simulink model "S2_VCO"  (Simulink 7.9)
settings: Solver=ode3  StartTime=0.0  StopTime=5.999  FixedStep=1/fs  RelTol=1e-3
values from neighbouring files (symbols this model uses):
  fs = fs/10    (= 100000)    [PLL_Parameter.m]
undefined symbols (not defined in the file or in its folder): get
libraries: dspspect3 x1, dspsigops x1, simulink x1, dspsnks4 x1
settings Model: Creator=Administrator  LastModifiedBy=root
settings DebuggingCC: FcnCallInpInsideContextMsg=Use local settings
settings GRTTargetCC: CombineOutputUpdateFcns=off  GRTInterface=on

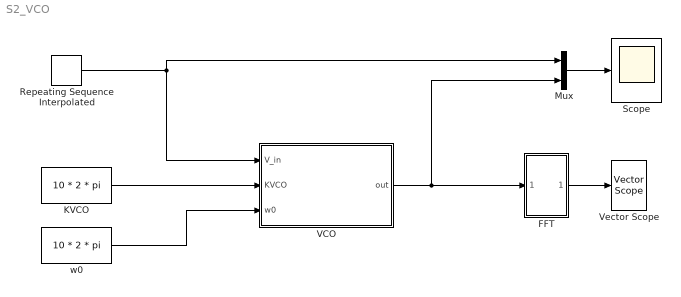
== system S2_VCO ==
  FFT : Subsystem  mask{Buffer_Length=2^14, nfft=2^14}
      mask prompts: Buffer_Length "Buffer length?"; nfft "FFt length?"
  KVCO : Constant  Value=10 * 2 * pi
  Mux : Mux  Inputs=2
  Repeating Sequence Interpolated : simulink/Sources/Repeating Sequence Interpolated  OutValues=[0 0 1 1 -1 -0.9].'  TimeValues=[0 1 3 3.5 5 6].'  LookUpMeth=Interpolation-Use End Values  tsamp=1/fs  OutMin=[]  OutMax=[]  OutDataTypeStr=double  OutputDataTypeScalingMode=double  OutDataType=fixdt(0,8)  OutScaling=2^-10
  Scope : Scope
      settings: TimeRange=1  YMin=-2  YMax=2
  VCO : Subsystem
  Vector Scope : dspsnks4/Vector Scope  ScopeProperties=on  Domain=Frequency  HorizSpan=1  DisplayProperties=off  AxisGrid=on  Memory=off  FrameNumber=on  AxisLegend=off  AxisZoom=off  OpenScopeAtSimStart=on  OpenScopeImmediately=off  FigPos=get(0,'defaultfigureposition')  AxisProperties=off  XUnits=Hertz  XRange=[0...Fs/2]  InheritXIncr=on  XIncr=1  XLabel=Time  XLimit=User-defined  XMin=0  XMax=30  XStart=0  YUnits=dB  YLabel=Amplitude  LineProperties=off  XAxisParamsVer=6.9
      settings: YMin=-100  YMax=100
  w0 : Constant  Value=10 * 2 * pi
  wires:
  VCO/1(out) -> Mux/2, FFT/1(In1)
  w0/1 -> VCO/3(w0)
  KVCO/1 -> VCO/2(KVCO)
  FFT/1(Out1) -> Vector Scope/1
  Repeating Sequence Interpolated/1 -> VCO/1(V_in), Mux/1
  Mux/1 -> Scope/1

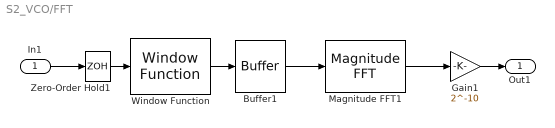
== system S2_VCO/FFT ==
  In1 : Inport
  Buffer1 : Buffer  N=Buffer_Length  TreatMby1Signals=One channel
  Gain1 : Gain  Gain=2^-10
  Magnitude FFT1 : dspspect3/Magnitude FFT  mag_or_magsq=Magnitude squared  FFTImplementation=Auto  fftLenInherit=off  fftsize=nfft
  Window Function : dspsigops/Window Function  winmode=Apply window to input  wintype=Blackman  sampmode=Continuous  samptime=1  N=64  Rs=50  beta=10  winsamp=Symmetric  UserWindow=hamming  OptParams=off  UserParams={'symmetric'}  RowConvenienceOn=on  dataType=double  isSigned=on  wordLen=16  udDataType=sfix(16)  fracBitsMode=Best precision  numFracBits=15  roundingMode=Floor  overflowMode=off  numSidelobes=4  sidelobeLevel=-30
  Zero-Order Hold1 : ZeroOrderHold  SampleTime=1/fs
  Out1 : Outport
  wires:
  Zero-Order Hold1/1 -> Window Function/1
  Buffer1/1 -> Magnitude FFT1/1
  Magnitude FFT1/1 -> Gain1/1
  Window Function/1 -> Buffer1/1
  In1/1 -> Zero-Order Hold1/1
  Gain1/1 -> Out1/1

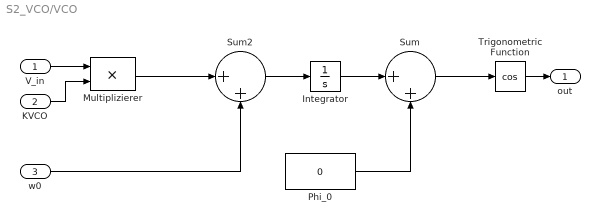
== system S2_VCO/VCO ==
  V_in : Inport
  KVCO : Inport  Port=2
  w0 : Inport  Port=3
  Integrator : Integrator
  Multiplizierer : Product  SaturateOnIntegerOverflow=on  RndMeth=Zero  InputSameDT=on  OutDataTypeStr=Inherit: Same as first input
  Phi_0 : Constant  Value=0
  Sum : Sum  Inputs=|++  SaturateOnIntegerOverflow=on  InputSameDT=on  OutDataTypeStr=Inherit: Same as first input
  Sum2 : Sum  Inputs=|++  SaturateOnIntegerOverflow=on  InputSameDT=on  OutDataTypeStr=Inherit: Same as first input
  Trigonometric Function : Trigonometry  Operator=cos
  out : Outport
  wires:
  w0/1 -> Sum2/2
  Sum/1 -> Trigonometric Function/1
  Integrator/1 -> Sum/1
  V_in/1 -> Multiplizierer/1
  Trigonometric Function/1 -> out/1
  Multiplizierer/1 -> Sum2/1
  Sum2/1 -> Integrator/1
  Phi_0/1 -> Sum/2
  KVCO/1 -> Multiplizierer/2
